simulink model "sim_tcyb_2024_att_ctrl"  (R2020a)
settings: Solver=ode4  StartTime=0.0  StopTime=30.0  FixedStep=0.01  RelTol=1e-3
values from neighbouring files (symbols this model uses):
  c1_diff_sigma_bar_w = diag([12; 12; 12])    [init_tcyb_2024_att_ctrl.m]
  c1_diff_ui = diag([25; 30; 20])    [init_tcyb_2024_att_ctrl.m]
  c2_diff_sigma_bar_w = diag([12; 12; 12])    [init_tcyb_2024_att_ctrl.m]
  c2_diff_ui = diag([50; 50; 10])    [init_tcyb_2024_att_ctrl.m]
  c3_diff_sigma_bar_w = diag([15; 15; 15])    [init_tcyb_2024_att_ctrl.m]
  c3_diff_ui = diag([15; 15; 10])    [init_tcyb_2024_att_ctrl.m]
  dw_aa_t = 0.2 * ones(3, 5) + ( 1.0 - 0.2 ) * rand(3, 5)    [init_tcyb_2024_att_ctrl.m]
  dw_ff_t = [ 0.4 * ones(1, 5) + ( 1.0 - 0.4 ) * rand(1, 5);                      0.4 * ones(1, 5) + ( 1.0 - 0.4 ) * rand(1, 5);                      0.2 * ones(1, 5) + ( 0.6 - 0.2 ) * rand(1, 5) ]    [init_tcyb_2024_att_ctrl.m]
  dw_phi_t = ( - pi / 2 ) * ones(3, 5) + ( pi / 2 - ( - pi / 2 ) ) * rand(3, 5)    [init_tcyb_2024_att_ctrl.m]
  dwci_init = zeros(3,NF)    [init_tcyb_2024_att_ctrl.m]
  h1w = diag([20.0; 20.0; 20.0])    [init_tcyb_2024_att_ctrl.m]
  h2w = diag([30.0; 35.0; 35.0])    [init_tcyb_2024_att_ctrl.m]
  h3w = diag([30.0; 25.0; 30.0])    [init_tcyb_2024_att_ctrl.m]
  Ji = zeros(3,3,NF)    [init_tcyb_2024_att_ctrl.m]
  ksg = diag([10.0, 10.0, 8.0])    [init_tcyb_2024_att_ctrl.m]
  kw = diag([10.0, 10.0, 8.0])    [init_tcyb_2024_att_ctrl.m]
  l1 = diag([5.0, 5.0, 4.0])    [init_tcyb_2024_att_ctrl.m]
  l2 = diag([5.0, 5.0, 4.0])    [init_tcyb_2024_att_ctrl.m]
  Lamd_diff_sigma_bar_w = 0.8    [init_tcyb_2024_att_ctrl.m]
  Lamd_diff_ui = 0.8    [init_tcyb_2024_att_ctrl.m]
  mu = diag([10.0, 10.0, 10.0, 8.0, 8.0, 8.0])    [init_tcyb_2024_att_ctrl.m]
  mu_d_w = 100    [init_tcyb_2024_att_ctrl.m]
  pos0 = zeros(3, 1)    [init_tcyb_2024_att_ctrl.m]
  PZ0 = P0(3)    [init_tcyb_2024_att_ctrl.m]
  PZ1 = 10    [init_tcyb_2024_att_ctrl.m]
  R0 = 4    [init_tcyb_2024_att_ctrl.m]
  R1 = 8    [init_tcyb_2024_att_ctrl.m]
  Rei_init = zeros(3,3,NF)    [init_tcyb_2024_att_ctrl.m]
  Ri_init = zeros(3,3,NF)    [init_tcyb_2024_att_ctrl.m]
  Rx2 = 10    [init_tcyb_2024_att_ctrl.m]
  Ry2 = 6    [init_tcyb_2024_att_ctrl.m]
  Rz2 = 4    [init_tcyb_2024_att_ctrl.m]
  sgei_init = zeros(3,NF)    [init_tcyb_2024_att_ctrl.m]
  sgi_init = zeros(3,NF)    [init_tcyb_2024_att_ctrl.m]
  T0 = 0    [init_tcyb_2024_att_ctrl.m]
  T1 = tseq1    (= 10)    [init_tcyb_2024_att_ctrl.m]
  T2 = tseq1 + tseq12 + tseq2    (= 30)    [init_tcyb_2024_att_ctrl.m]
  ui_init = zeros(3,NF)    [init_tcyb_2024_att_ctrl.m]
  V_Phi_Rei_init = zeros(3,NF)    [init_tcyb_2024_att_ctrl.m]
  vel0 = zeros(3, 1)    [init_tcyb_2024_att_ctrl.m]
  wci_init = zeros(3,NF)    [init_tcyb_2024_att_ctrl.m]
  wei_init = zeros(3,NF)    [init_tcyb_2024_att_ctrl.m]
  zeta_diff_sigma_bar_w = 0.3    [init_tcyb_2024_att_ctrl.m]
  zeta_diff_ui = 0.05    [init_tcyb_2024_att_ctrl.m]
undefined symbols (not defined in the file or in its folder): cal_frac_squ, p_alfaw1, p_alfaw2, q_alfaw1, q_alfaw2, wi_init
(part 5 of 5)

== matlab function sim_tcyb_2024_att_ctrl/trans to column16 ==
  data: x input; y output
function y = fcn(x)
y = x(:);

== matlab function sim_tcyb_2024_att_ctrl/cal d_theta_hat2 ==
  data: c1 input; d_ui_hat output; d_dui_hat output; d_d2ui_hat output; c2 input; c3 input; chi_t input; ui_sig_1 input; ui_sig_2 input; ui_sig_3 input; ui_sig_4 input; ui_sig_5 input; ui_sig_6 input; dui_hat input; d2ui_hat input
function [d_ui_hat, d_dui_hat, d_d2ui_hat] = fcn(c1, c2, c3, chi_t, ui_sig_1, ui_sig_2, ui_sig_3, ...
                                                                                        ui_sig_4, ui_sig_5, ui_sig_6, dui_hat, d2ui_hat)
d_d2ui_hat = -chi_t .* c1 * ui_sig_1(:) - (1 - chi_t) .* c1 * ui_sig_2(:);
d_dui_hat = -chi_t .* c2 * ui_sig_3(:) - (1 - chi_t) .* c2 * ui_sig_4(:) + d2ui_hat(:);
d_ui_hat = -chi_t .* c3 * ui_sig_5(:) - (1 - chi_t) .* c3 * ui_sig_6(:) + dui_hat(:);

== matlab function sim_tcyb_2024_att_ctrl/cal sig12 ==
  data: x input; z output; y input
function z = fcn(x, y)
z = x(:) .* sign(y(:));

== matlab function sim_tcyb_2024_att_ctrl/cal sig13 ==
  data: x input; z output; y input
function z = fcn(x, y)
z = x(:) .* sign(y(:));

== matlab function sim_tcyb_2024_att_ctrl/cal sig14 ==
  data: x input; z output; y input
function z = fcn(x, y)
z = x(:) .* sign(y(:));

== matlab function sim_tcyb_2024_att_ctrl/cal sig15 ==
  data: x input; z output; y input
function z = fcn(x, y)
z = x(:) .* sign(y(:));

== matlab function sim_tcyb_2024_att_ctrl/cal sig16 ==
  data: x input; z output; y input
function z = fcn(x, y)
z = x(:) .* sign(y(:));

== matlab function sim_tcyb_2024_att_ctrl/cal sig17 ==
  data: x input; z output; y input
function z = fcn(x, y)
z = x(:) .* sign(y(:));

== matlab function sim_tcyb_2024_att_ctrl/choose ui agent 3 ==
  data: x input; y output
function y = fcn(x)
iiuav = 3;
y = x(:,iiuav);

== matlab function sim_tcyb_2024_att_ctrl/trans to column17 ==
  data: x input; y output
function y = fcn(x)
y = x(:);

== matlab function sim_tcyb_2024_att_ctrl/trans to column18 ==
  data: x input; y output
function y = fcn(x)
y = x(:);

== matlab function sim_tcyb_2024_att_ctrl/trans to column19 ==
  data: x input; y output
function y = fcn(x)
y = x(:);

== matlab function sim_tcyb_2024_att_ctrl/trans to column20 ==
  data: x input; y output
function y = fcn(x)
y = x(:);

== matlab function sim_tcyb_2024_att_ctrl/trans to column21 ==
  data: x input; y output
function y = fcn(x)
y = x(:);

== matlab function sim_tcyb_2024_att_ctrl/trans to column22 ==
  data: x input; y output
function y = fcn(x)
y = x(:);

== matlab function sim_tcyb_2024_att_ctrl/cal d_theta_hat3 ==
  data: c1 input; d_ui_hat output; d_dui_hat output; d_d2ui_hat output; c2 input; c3 input; chi_t input; ui_sig_1 input; ui_sig_2 input; ui_sig_3 input; ui_sig_4 input; ui_sig_5 input; ui_sig_6 input; dui_hat input; d2ui_hat input
function [d_ui_hat, d_dui_hat, d_d2ui_hat] = fcn(c1, c2, c3, chi_t, ui_sig_1, ui_sig_2, ui_sig_3, ...
                                                                                        ui_sig_4, ui_sig_5, ui_sig_6, dui_hat, d2ui_hat)
d_d2ui_hat = -chi_t .* c1 * ui_sig_1(:) - (1 - chi_t) .* c1 * ui_sig_2(:);
d_dui_hat = -chi_t .* c2 * ui_sig_3(:) - (1 - chi_t) .* c2 * ui_sig_4(:) + d2ui_hat(:);
d_ui_hat = -chi_t .* c3 * ui_sig_5(:) - (1 - chi_t) .* c3 * ui_sig_6(:) + dui_hat(:);

== matlab function sim_tcyb_2024_att_ctrl/cal sig18 ==
  data: x input; z output; y input
function z = fcn(x, y)
z = x(:) .* sign(y(:));

== matlab function sim_tcyb_2024_att_ctrl/cal Gamma_wi agent 2 ==
  data: wi_vec input; Gamma_wi_2 output
function Gamma_wi_2 = fcn(wi_vec)
%%%% 计算矩阵 Gamma_wi
iiuav = 2;
Gamma_wi_2 = [wi_vec(1,iiuav), 0, 0, 0, wi_vec(3,iiuav), wi_vec(2,iiuav); ...
                                0, wi_vec(2,iiuav), 0, wi_vec(3,iiuav), 0, wi_vec(1,iiuav); ...
                                0, 0, wi_vec(3,iiuav), wi_vec(2,iiuav), wi_vec(1,iiuav), 0];
end

== matlab function sim_tcyb_2024_att_ctrl/cal sig19 ==
  data: x input; z output; y input
function z = fcn(x, y)
z = x(:) .* sign(y(:));

== matlab function sim_tcyb_2024_att_ctrl/cal sig20 ==
  data: x input; z output; y input
function z = fcn(x, y)
z = x(:) .* sign(y(:));

== matlab function sim_tcyb_2024_att_ctrl/cal sig21 ==
  data: x input; z output; y input
function z = fcn(x, y)
z = x(:) .* sign(y(:));

== matlab function sim_tcyb_2024_att_ctrl/cal sig22 ==
  data: x input; z output; y input
function z = fcn(x, y)
z = x(:) .* sign(y(:));

== matlab function sim_tcyb_2024_att_ctrl/cal sig23 ==
  data: x input; z output; y input
function z = fcn(x, y)
z = x(:) .* sign(y(:));

== matlab function sim_tcyb_2024_att_ctrl/choose ui agent 4 ==
  data: x input; y output
function y = fcn(x)
iiuav = 4;
y = x(:,iiuav);

== matlab function sim_tcyb_2024_att_ctrl/trans to column23 ==
  data: x input; y output
function y = fcn(x)
y = x(:);

== matlab function sim_tcyb_2024_att_ctrl/trans to column24 ==
  data: x input; y output
function y = fcn(x)
y = x(:);

== matlab function sim_tcyb_2024_att_ctrl/process velocity ==
  data: T0 input; T1 input; T2 input; PZ0 input; PZ1 input; R0 input; R1 input; Rx2 input; Ry2 input; Rz2 input; t input; V_init_out output
function V_init_out = fcn(T0, T1, T2, PZ0, PZ1, R0, R1, Rx2, Ry2, Rz2, t)
V_init_out = zeros(3, 1);
if t < T1 + 1e-05
    V_init_out(1, 1) = ( cos( ( 2 * pi * ( t - T0 ) ) / ( T0 - T1 ) ) * ( R0 - R1 ) ) / ( T0 - T1 ) ...
                                    - ( 2 * pi * sin( ( 2 * pi * ( t - T0 ) ) / ( T0 - T1 ) ) * ( R0 + ( ( R0 - R1 ) * ( t - T0 ) ) / ( T0 - T1 ) ) ) / ( T0 - T1 );
    V_init_out(2, 1) = ( sin( ( 2 * pi * ( t - T0 ) ) / ( T0 - T1 ) ) * ( R0 - R1 ) ) / ( T0 - T1 ) ...
                                    + ( 2 * pi * cos( ( 2 * pi * ( t - T0 ) ) / ( T0 - T1 ) ) * ( R0 + ( ( R0 - R1 ) * ( t - T0 ) ) / ( T0 - T1 ) ) ) / ( T0 - T1 );
    V_init_out(3, 1) = ( PZ0 - PZ1 ) / ( T0 - T1 );
else
    V_init_out(1, 1) = ( 2 * Rx2 * pi * sin( ( 2 * pi * ( t - T1 ) ) / ( T1 - T2 ) ) ) / ( T1 - T2 );
    V_init_out(2, 1) = ( 4 * Ry2 * pi * cos( ( 4 * pi * ( t - T1 ) ) / ( T1 - T2 ) ) ) / ( T1 - T2 );
    V_init_out(3, 1) = - ( 4 * Rz2 * pi * cos( ( 4 * pi * ( t - T1 ) ) / ( T1 - T2 ) ) ) / ( T1 - T2 );
end

== matlab function sim_tcyb_2024_att_ctrl/trans to column25 ==
  data: x input; y output
function y = fcn(x)
y = x(:);

== matlab function sim_tcyb_2024_att_ctrl/trans to column26 ==
  data: x input; y output
function y = fcn(x)
y = x(:);

== matlab function sim_tcyb_2024_att_ctrl/trans to column27 ==
  data: x input; y output
function y = fcn(x)
y = x(:);

== matlab function sim_tcyb_2024_att_ctrl/trans to column28 ==
  data: x input; y output
function y = fcn(x)
y = x(:);

== matlab function sim_tcyb_2024_att_ctrl/cal d_theta_hat4 ==
  data: c1 input; d_ui_hat output; d_dui_hat output; d_d2ui_hat output; c2 input; c3 input; chi_t input; ui_sig_1 input; ui_sig_2 input; ui_sig_3 input; ui_sig_4 input; ui_sig_5 input; ui_sig_6 input; dui_hat input; d2ui_hat input
function [d_ui_hat, d_dui_hat, d_d2ui_hat] = fcn(c1, c2, c3, chi_t, ui_sig_1, ui_sig_2, ui_sig_3, ...
                                                                                        ui_sig_4, ui_sig_5, ui_sig_6, dui_hat, d2ui_hat)
d_d2ui_hat = -chi_t .* c1 * ui_sig_1(:) - (1 - chi_t) .* c1 * ui_sig_2(:);
d_dui_hat = -chi_t .* c2 * ui_sig_3(:) - (1 - chi_t) .* c2 * ui_sig_4(:) + d2ui_hat(:);
d_ui_hat = -chi_t .* c3 * ui_sig_5(:) - (1 - chi_t) .* c3 * ui_sig_6(:) + dui_hat(:);

== matlab function sim_tcyb_2024_att_ctrl/cal sig24 ==
  data: x input; z output; y input
function z = fcn(x, y)
z = x(:) .* sign(y(:));

== matlab function sim_tcyb_2024_att_ctrl/cal sig25 ==
  data: x input; z output; y input
function z = fcn(x, y)
z = x(:) .* sign(y(:));

== matlab function sim_tcyb_2024_att_ctrl/cal sig26 ==
  data: x input; z output; y input
function z = fcn(x, y)
z = x(:) .* sign(y(:));

== matlab function sim_tcyb_2024_att_ctrl/cal sig27 ==
  data: x input; z output; y input
function z = fcn(x, y)
z = x(:) .* sign(y(:));

== matlab function sim_tcyb_2024_att_ctrl/cal sig28 ==
  data: x input; z output; y input
function z = fcn(x, y)
z = x(:) .* sign(y(:));

== matlab function sim_tcyb_2024_att_ctrl/cal sig29 ==
  data: x input; z output; y input
function z = fcn(x, y)
z = x(:) .* sign(y(:));

== matlab function sim_tcyb_2024_att_ctrl/choose ui agent 5 ==
  data: x input; y output
function y = fcn(x)
iiuav = 5;
y = x(:,iiuav);

== matlab function sim_tcyb_2024_att_ctrl/trans to column29 ==
  data: x input; y output
function y = fcn(x)
y = x(:);

== matlab function sim_tcyb_2024_att_ctrl/trans to column30 ==
  data: x input; y output
function y = fcn(x)
y = x(:);

== matlab function sim_tcyb_2024_att_ctrl/trans to column31 ==
  data: x input; y output
function y = fcn(x)
y = x(:);

== matlab function sim_tcyb_2024_att_ctrl/trans to column32 ==
  data: x input; y output
function y = fcn(x)
y = x(:);

== matlab function sim_tcyb_2024_att_ctrl/trans to column33 ==
  data: x input; y output
function y = fcn(x)
y = x(:);

== matlab function sim_tcyb_2024_att_ctrl/trans to column34 ==
  data: x input; y output
function y = fcn(x)
y = x(:);
